simulink model "spring_ball"  (Simulink 4.00)
settings: Solver=ode45  SolverMode=SingleTasking  StartTime=0.0  StopTime=10.0  FixedStep=0.001  MaxStep=0.01  RelTol=1e-3
undefined symbols (not defined in the file or in its folder): Stossvelocity
libraries: simulink3 x1
settings Model: LastModifiedBy=Brunner  LimitDataPoints=off  RTWOptions="-aExtMode=0 -aForceParamTrailComments=0 -aInlineInvariantSignals=0 -aLocalBlockOutputs=1 -aLogVarNameModifier=\"rt_\" -aRTWVerbose=1 -aRollThreshold=5 -aShowEliminatedStatements=1"  BlockReductionOpt=off

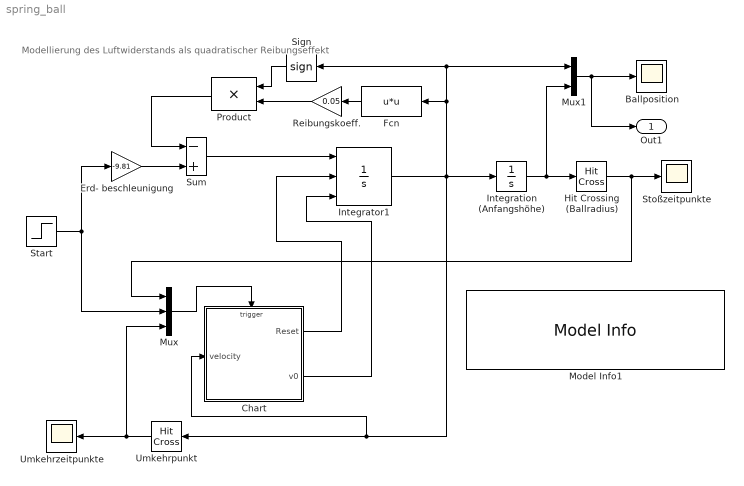
== system spring_ball ==
  note: Modellierung des Luftwiderstands
      | als quadratischer Reibungseffekt
  Ballposition : Scope
      settings: TimeRange=auto  YMin=-5  YMax=5  SaveToWorkspace=off  SaveName=ScopeData  LimitDataPoints=on  MaxDataPoints=5000
  Chart : Stateflow chart  TreatAsAtomicUnit=on
      settings: RTWFcnNameOpts=Auto  RTWFileNameOpts=Auto
  Erd- beschleunigung : Gain  Gain=-9.81  Multiplication=Element-wise(K.*u)  SaturateOnIntegerOverflow=on
  Fcn : Fcn  Orientation=left  Expr=u*u
  Hit Crossing (Ballradius) : HitCross  HitCrossingOffset=0.1  HitCrossingDirection=falling  ShowOutputPort=on
  Integration (Anfangshöhe) : Integrator  ExternalReset=none  InitialConditionSource=internal  InitialCondition=5  LimitOutput=off  UpperSaturationLimit=inf  LowerSaturationLimit=-inf  ShowSaturationPort=off  ShowStatePort=off  AbsoluteTolerance=auto
  Integrator1 : Integrator  ExternalReset=rising  InitialConditionSource=external  InitialCondition=Stossvelocity  LimitOutput=off  UpperSaturationLimit=inf  LowerSaturationLimit=-inf  ShowSaturationPort=off  ShowStatePort=off  AbsoluteTolerance=auto
  Model Info1 : simulink3/Signals & Systems/Model Info  InitialBlockCM=none  BlockCM=none  Frame=on  DisplayStringWithTags=|  HorizontalTextAlignment=Center  LeftAlignmentValue=0.5  SourceBlockDiagram=spring_ball_alt  TagMaxNumber=20
      | Modell eines auf einer Fläche springenden Balls
      | (Annahme:  elastischer Stoß)
  Mux : Mux  Inputs=3
  Mux1 : Mux  Inputs=2
  Product : Product  Orientation=left  Inputs=2  Multiplication=Element-wise(.*)  SaturateOnIntegerOverflow=on
  Reibungskoeff. : Gain  Orientation=left  Gain=0.05  Multiplication=Element-wise(K.*u)  SaturateOnIntegerOverflow=on
  Sign : Signum  Orientation=left
  Start : Step  Time=1  Before=0  After=1  SampleTime=0
  Stoßzeitpunkte : Scope
      settings: TimeRange=auto  YMin=-5  YMax=5  SaveToWorkspace=off  LimitDataPoints=on  MaxDataPoints=5000
  Sum : Sum  Inputs=-+  SaturateOnIntegerOverflow=on
  Umkehrpunkt : HitCross  Orientation=left  HitCrossingOffset=0  HitCrossingDirection=falling  ShowOutputPort=on
  Umkehrzeitpunkte : Scope
      settings: TimeRange=auto  YMin=-5  YMax=5  SaveToWorkspace=off  SaveName=ScopeData2  LimitDataPoints=on  MaxDataPoints=5000
  Out1 : Outport  Port=1
  wires:
  Fcn/1 -> Reibungskoeff./1
  Hit Crossing (Ballradius)/1 -> Mux/1, Stoßzeitpunkte/1
  Start/1 -> Erd- beschleunigung/1, Mux/2
  Sum/1 -> Integrator1/1
  Integrator1/1 -> Integration (Anfangshöhe)/1, Fcn/1, Mux1/1, Sign/1, Umkehrpunkt/1, Chart/1(velocity)
  Integration (Anfangshöhe)/1 -> Hit Crossing (Ballradius)/1, Mux1/2
  Mux1/1 -> Ballposition/1, Out1/1
  Chart/1(Reset) -> Integrator1/2
  Chart/2(v0) -> Integrator1/3
  Reibungskoeff./1 -> Product/2
  Sign/1 -> Product/1
  Product/1 -> Sum/1
  Erd- beschleunigung/1 -> Sum/2
  Mux/1 -> Chart/Trigger
  Umkehrpunkt/1 -> Mux/3, Umkehrzeitpunkte/1

== stateflow chart Chart ==
  state Ball_fallend/
    entry:Reset=0;
    v0=0;
  state Ball_steigend/
    entry: v0=-velocity;
    Reset=1;
  (default) -> Ball_fallend
  Ball_fallend -> Ball_steigend : Aufprall
  Ball_steigend -> Ball_fallend : Umkehr
  data: Reset output double; v0 output double; velocity input double
  events: Aufprall input RISING_EDGE_EVENT; Enable input EITHER_EDGE_EVENT; Umkehr input RISING_EDGE_EVENT
